simulink subsystem "Sensor"  (R2023b)
settings: Solver=VariableStepAuto  StartTime=0.0  StopTime=10.0  RelTol=1e-3
libraries: arduinolib x2
settings Model: Creator=chaya  LastModifiedBy=chaya

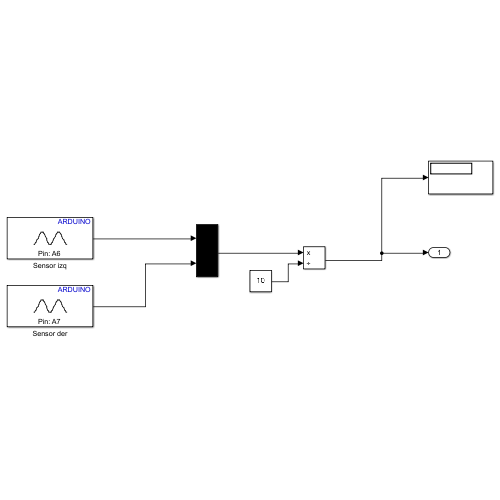
[thumbnail: Simulink's stored preview of the top-level diagram]
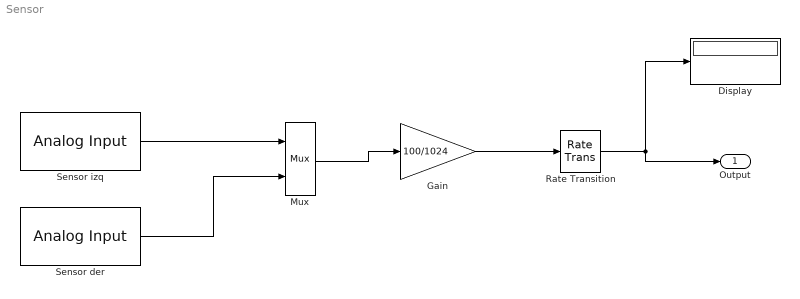
== system Sensor ==
  Display : Display
  Gain : Gain  Gain=100/1024  OutDataTypeStr=uint16
  Mux : Mux  Inputs=2
  Rate Transition : RateTransition
  Sensor der : arduinolib/Analog Input  pinNumber=6  ReadResultsOnly=off  ConversionTriggerSource=Software  ExternalTriggerType=uint32( 0 )  OutputDataType=uint16  EnableConversionCompleteNotify=off  EnableOuputStatus=off  SampleTime=0.05  blockPlatform=arduino
  Sensor izq : arduinolib/Analog Input  pinNumber=7  ReadResultsOnly=off  ConversionTriggerSource=Software  ExternalTriggerType=uint32( 0 )  OutputDataType=uint16  EnableConversionCompleteNotify=off  EnableOuputStatus=off  SampleTime=0.05  blockPlatform=arduino
  Output : Outport
  wires:
  Mux/1 -> Gain/1
  Sensor izq/1 -> Mux/1
  Sensor der/1 -> Mux/2
  Rate Transition/1 -> Display/1, Output/1
  Gain/1 -> Rate Transition/1
